simulink model "bo1808_foc_svpwm_bo1808"  (R2024b)
settings: Solver=ode23tb  StartTime=0.0  StopTime=t_stop_position_loop  MaxStep=Ts_sim_foc_svpwm  RelTol=1e-3
PostLoadFcn:
  | try, mf=get_param(bdroot,'FileName'); if ~isempty(mf), addpath(fileparts(fileparts(mf))); end, catch, end
InitFcn:
  | try, mf=get_param(bdroot,'FileName'); if ~isempty(mf), addpath(fileparts(fileparts(mf))); end, catch, end
model workspace (MAT data in the model file):
  B = 5.1285732711e-07
  Id_max = 0.6
  Iq_max = 0.25
  J = 1.4e-07
  Ki_id = 13571.6802635
  Ki_iq = 13571.6802635
  Ki_w = 0.279803284771
  Kp_id = 0.697433569097
  Kp_iq = 0.697433569097
  Kp_pos = 37.6991118431
  Kp_w = 0.0043730736291
  Kt_q = 0.0064
  Ld = 0.00037
  Lq = 0.00037
  Rs = 7.2
  TL_amp_sine = 0.0004
  TL_load_mode = 'step'
  TL_mean_sine = 0.0012
  TL_noise_enable = 0
  TL_noise_sample_time = 0.0001
  TL_noise_seed = 1808
  TL_noise_std = 5e-05
  TL_nom = 0.0012
  TL_sine_start = 0.12
  TL_step_time_fig3_9 = 0.12
  Ts_pwm = 2e-05
  Ts_sim_foc_svpwm = 2e-06
  Vdc = 11.4
  Vdq_max = 6.58179306876
  f_load_sine = 50
  foc_control_mode = 'position'
  omega_ref_pos_max = 104.71975512
  pn = 4
  position_ref_step_time = 0.005
  psi_f = 0.00106666666667
  speed_ref_fig3_9_rpm = 1000
  t_stop_foc_svpwm = 0.25
  t_stop_position_loop = 0.4
  theta_e0 = 0
  theta_m0 = 0
  theta_m_ref_step = 0.523598775598
libraries: simulink x1
settings Model: Creator=26683  LastModifiedBy=26683

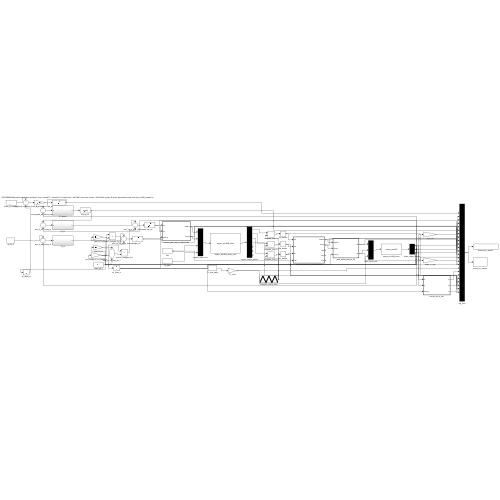
[thumbnail: Simulink's stored preview of the top-level diagram]
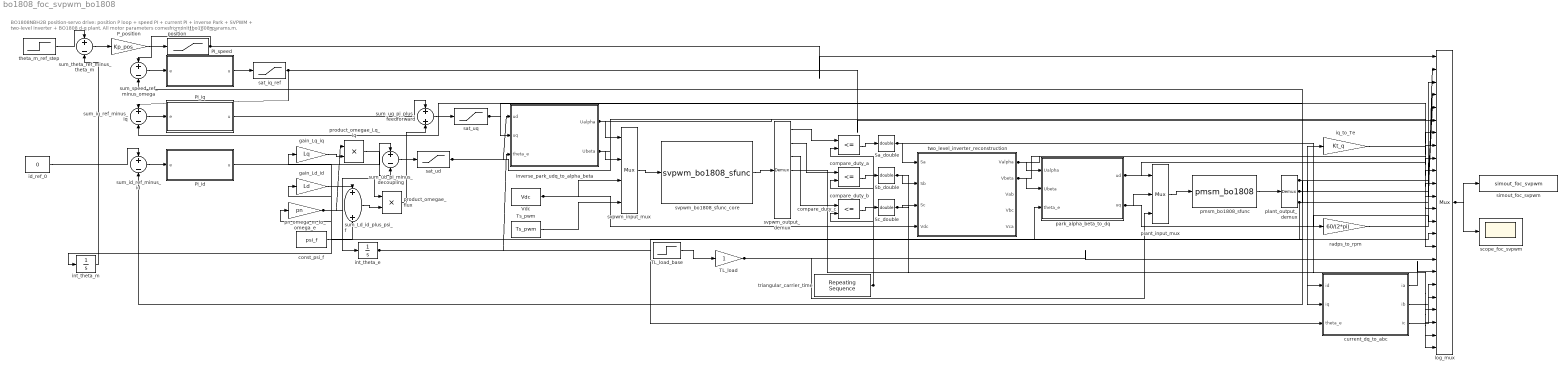
== system bo1808_foc_svpwm_bo1808 ==
  note: BO1808NBH2B position-servo drive: position P loop + speed PI + current PI + inverse Park + SVPWM + two-level inverter + BO1808 d-q plant. All motor parameters come from init_bo1808_params.m.
  PI_id : Subsystem
  PI_iq : Subsystem
  PI_speed : Subsystem
  P_position : Gain  Gain=Kp_pos
  Sa_double : DataTypeConversion  OutDataTypeStr=double  SaturateOnIntegerOverflow=off  RndMeth=Floor
  Sb_double : DataTypeConversion  OutDataTypeStr=double  SaturateOnIntegerOverflow=off  RndMeth=Floor
  Sc_double : DataTypeConversion  OutDataTypeStr=double  SaturateOnIntegerOverflow=off  RndMeth=Floor
  TL_load : Gain
  TL_load_base : Step  Time=TL_step_time_fig3_9  After=TL_nom  SampleTime=0
  Ts_pwm : Constant  Value=Ts_pwm
  Vdc : Constant  Value=Vdc
  compare_duty_a : RelationalOperator  Operator=<=  OutDataTypeStr=boolean  RndMeth=Simplest  InputSameDT=off
  compare_duty_b : RelationalOperator  Operator=<=  OutDataTypeStr=boolean  RndMeth=Simplest  InputSameDT=off
  compare_duty_c : RelationalOperator  Operator=<=  OutDataTypeStr=boolean  RndMeth=Simplest  InputSameDT=off
  const_psi_f : Constant  Value=psi_f
  current_dq_to_abc : MATLAB Function  TreatAsAtomicUnit=on
  gain_Ld_id : Gain  Gain=Ld
  gain_Lq_iq : Gain  Gain=Lq
  id_ref_0 : Constant  Value=0
  int_theta_e : Integrator  InitialCondition=theta_e0
  int_theta_m : Integrator  InitialCondition=theta_m0
  inverse_park_udq_to_alpha_beta : MATLAB Function  TreatAsAtomicUnit=on
  iq_to_Te : Gain  Gain=Kt_q
  log_mux : Mux  Inputs=24
  park_alpha_beta_to_dq : MATLAB Function  TreatAsAtomicUnit=on
  plant_input_mux : Mux  Inputs=3
  plant_output_demux : Demux  Outputs=3
  pmsm_bo1808_sfunc : S-Function  FunctionName=pmsm_bo1808  SFunctionDeploymentMode=off  EnableBusSupport=off
  pn_omega_m_to_omega_e : Gain  Gain=pn
  product_omegae_Lq_iq : Product  Inputs=**
  product_omegae_flux : Product  Inputs=**
  radps_to_rpm : Gain  Gain=60/(2*pi)
  sat_iq_ref : Saturate  UpperLimit=Iq_max  LowerLimit=-Iq_max
  sat_speed_ref_from_position : Saturate  UpperLimit=omega_ref_pos_max  LowerLimit=-omega_ref_pos_max
  sat_ud : Saturate  UpperLimit=Vdq_max  LowerLimit=-Vdq_max
  sat_uq : Saturate  UpperLimit=Vdq_max  LowerLimit=-Vdq_max
  scope_foc_svpwm : Scope
  simout_foc_svpwm : ToWorkspace  VariableName=simout_foc_svpwm  SaveFormat=Structure With Time  SampleTime=-1
  sum_Ld_id_plus_psi_f : Sum
  sum_id_ref_minus_id : Sum  Inputs=+-
  sum_iq_ref_minus_iq : Sum  Inputs=+-
  sum_speed_ref_minus_omega : Sum  Inputs=+-
  sum_theta_ref_minus_theta_m : Sum  Inputs=+-
  sum_ud_pi_minus_decoupling : Sum  Inputs=+-
  sum_uq_pi_plus_feedforward : Sum
  svpwm_bo1808_sfunc_core : S-Function  FunctionName=svpwm_bo1808_sfunc  SFunctionDeploymentMode=off  EnableBusSupport=off
  svpwm_input_mux : Mux
  svpwm_output_demux : Demux  Outputs=7
  theta_m_ref_step : Step  Time=position_ref_step_time  After=theta_m_ref_step  SampleTime=0
  triangular_carrier_time : simulink/Sources/Repeating Sequence  rep_seq_t=[0 Ts_pwm/2 Ts_pwm]  rep_seq_y=[0 Ts_pwm/2 0]
  two_level_inverter_reconstruction : MATLAB Function  TreatAsAtomicUnit=on
  wires:
  TL_load_base/1 -> TL_load/1
  theta_m_ref_step/1 -> sum_theta_ref_minus_theta_m/1
  sum_theta_ref_minus_theta_m/1 -> P_position/1
  P_position/1 -> sat_speed_ref_from_position/1
  sat_speed_ref_from_position/1 -> sum_speed_ref_minus_omega/1, log_mux/1
  sum_speed_ref_minus_omega/1 -> PI_speed/1(e)
  PI_speed/1(u) -> sat_iq_ref/1
  sat_iq_ref/1 -> sum_iq_ref_minus_iq/1, log_mux/6
  id_ref_0/1 -> sum_id_ref_minus_id/1
  sum_iq_ref_minus_iq/1 -> PI_iq/1(e)
  sum_id_ref_minus_id/1 -> PI_id/1(e)
  PI_id/1(u) -> sum_ud_pi_minus_decoupling/1
  product_omegae_Lq_iq/1 -> sum_ud_pi_minus_decoupling/2
  sum_ud_pi_minus_decoupling/1 -> sat_ud/1
  PI_iq/1(u) -> sum_uq_pi_plus_feedforward/1
  product_omegae_flux/1 -> sum_uq_pi_plus_feedforward/2
  sum_uq_pi_plus_feedforward/1 -> sat_uq/1
  sat_ud/1 -> inverse_park_udq_to_alpha_beta/1(ud), log_mux/7
  sat_uq/1 -> inverse_park_udq_to_alpha_beta/2(uq), log_mux/8
  int_theta_e/1 -> inverse_park_udq_to_alpha_beta/3(theta_e), park_alpha_beta_to_dq/3(theta_e), current_dq_to_abc/3(theta_e), log_mux/15
  inverse_park_udq_to_alpha_beta/1(Ualpha) -> svpwm_input_mux/1, log_mux/9
  inverse_park_udq_to_alpha_beta/2(Ubeta) -> svpwm_input_mux/2, log_mux/10
  Vdc/1 -> svpwm_input_mux/3, two_level_inverter_reconstruction/4(Vdc)
  Ts_pwm/1 -> svpwm_input_mux/4
  svpwm_input_mux/1 -> svpwm_bo1808_sfunc_core/1
  svpwm_bo1808_sfunc_core/1 -> svpwm_output_demux/1
  svpwm_output_demux/1 -> compare_duty_a/1
  svpwm_output_demux/2 -> compare_duty_b/1
  svpwm_output_demux/3 -> compare_duty_c/1
  triangular_carrier_time/1 -> compare_duty_a/2, compare_duty_b/2, compare_duty_c/2
  compare_duty_a/1 -> Sa_double/1
  compare_duty_b/1 -> Sb_double/1
  compare_duty_c/1 -> Sc_double/1
  Sa_double/1 -> two_level_inverter_reconstruction/1(Sa), log_mux/22
  Sb_double/1 -> two_level_inverter_reconstruction/2(Sb), log_mux/23
  Sc_double/1 -> two_level_inverter_reconstruction/3(Sc), log_mux/24
  two_level_inverter_reconstruction/1(Valpha) -> park_alpha_beta_to_dq/1(Ualpha), log_mux/11
  two_level_inverter_reconstruction/2(Vbeta) -> park_alpha_beta_to_dq/2(Ubeta), log_mux/12
  park_alpha_beta_to_dq/1(ud) -> plant_input_mux/1, log_mux/13
  park_alpha_beta_to_dq/2(uq) -> plant_input_mux/2, log_mux/14
  TL_load/1 -> plant_input_mux/3, log_mux/17
  plant_input_mux/1 -> pmsm_bo1808_sfunc/1
  pmsm_bo1808_sfunc/1 -> plant_output_demux/1
  plant_output_demux/1 -> sum_id_ref_minus_id/2, gain_Ld_id/1, current_dq_to_abc/1(id), log_mux/4
  plant_output_demux/2 -> sum_iq_ref_minus_iq/2, iq_to_Te/1, gain_Lq_iq/1, current_dq_to_abc/2(iq), log_mux/5
  plant_output_demux/3 -> sum_speed_ref_minus_omega/2, int_theta_m/1, pn_omega_m_to_omega_e/1, radps_to_rpm/1, log_mux/2
  int_theta_m/1 -> sum_theta_ref_minus_theta_m/2
  pn_omega_m_to_omega_e/1 -> int_theta_e/1, product_omegae_Lq_iq/1, product_omegae_flux/1
  gain_Lq_iq/1 -> product_omegae_Lq_iq/2
  gain_Ld_id/1 -> sum_Ld_id_plus_psi_f/1
  const_psi_f/1 -> sum_Ld_id_plus_psi_f/2
  sum_Ld_id_plus_psi_f/1 -> product_omegae_flux/2
  radps_to_rpm/1 -> log_mux/3
  iq_to_Te/1 -> log_mux/16
  current_dq_to_abc/1(ia) -> log_mux/18
  current_dq_to_abc/2(ib) -> log_mux/19
  current_dq_to_abc/3(ic) -> log_mux/20
  svpwm_output_demux/4 -> log_mux/21
  log_mux/1 -> simout_foc_svpwm/1, scope_foc_svpwm/1

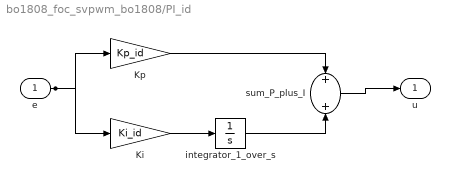
== system bo1808_foc_svpwm_bo1808/PI_id ==
  e : Inport
  Ki : Gain  Gain=Ki_id
  Kp : Gain  Gain=Kp_id
  integrator_1_over_s : Integrator
  sum_P_plus_I : Sum
  u : Outport
  wires:
  e/1 -> Kp/1, Ki/1
  Kp/1 -> sum_P_plus_I/1
  Ki/1 -> integrator_1_over_s/1
  integrator_1_over_s/1 -> sum_P_plus_I/2
  sum_P_plus_I/1 -> u/1

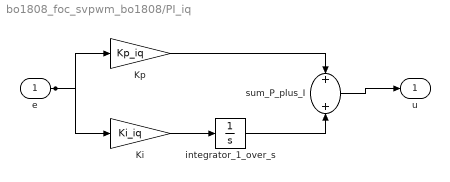
== system bo1808_foc_svpwm_bo1808/PI_iq ==
  e : Inport
  Ki : Gain  Gain=Ki_iq
  Kp : Gain  Gain=Kp_iq
  integrator_1_over_s : Integrator
  sum_P_plus_I : Sum
  u : Outport
  wires:
  e/1 -> Kp/1, Ki/1
  Kp/1 -> sum_P_plus_I/1
  Ki/1 -> integrator_1_over_s/1
  integrator_1_over_s/1 -> sum_P_plus_I/2
  sum_P_plus_I/1 -> u/1

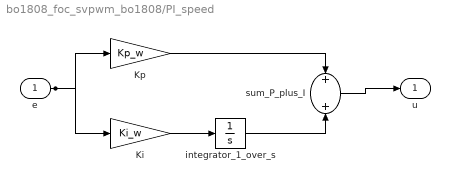
== system bo1808_foc_svpwm_bo1808/PI_speed ==
  e : Inport
  Ki : Gain  Gain=Ki_w
  Kp : Gain  Gain=Kp_w
  integrator_1_over_s : Integrator
  sum_P_plus_I : Sum
  u : Outport
  wires:
  e/1 -> Kp/1, Ki/1
  Kp/1 -> sum_P_plus_I/1
  Ki/1 -> integrator_1_over_s/1
  integrator_1_over_s/1 -> sum_P_plus_I/2
  sum_P_plus_I/1 -> u/1

== matlab function bo1808_foc_svpwm_bo1808/two_level_inverter_reconstruction ==
  data: Sa input; Valpha output; Sb input; Sc input; Vdc input; Vbeta output; Vab output; Vbc output; Vca output
function [Valpha,Vbeta,Vab,Vbc,Vca] = fcn(Sa,Sb,Sc,Vdc)
%#codegen
sa = double(Sa);
sb = double(Sb);
sc = double(Sc);
Va0 = (sa - 0.5)*Vdc;
Vb0 = (sb - 0.5)*Vdc;
Vc0 = (sc - 0.5)*Vdc;
Vab = Va0 - Vb0;
Vbc = Vb0 - Vc0;
Vca = Vc0 - Va0;
Valpha = (2/3)*(Va0 - 0.5*Vb0 - 0.5*Vc0);
Vbeta = (2/3)*(sqrt(3)/2)*(Vb0 - Vc0);
end

== matlab function bo1808_foc_svpwm_bo1808/inverse_park_udq_to_alpha_beta ==
  data: ud input; Ualpha output; uq input; theta_e input; Ubeta output
function [Ualpha,Ubeta] = fcn(ud,uq,theta_e)
%#codegen
c = cos(theta_e);
s = sin(theta_e);
Ualpha = ud*c - uq*s;
Ubeta = ud*s + uq*c;
end

== matlab function bo1808_foc_svpwm_bo1808/park_alpha_beta_to_dq ==
  data: Ualpha input; ud output; Ubeta input; theta_e input; uq output
function [ud,uq] = fcn(Ualpha,Ubeta,theta_e)
%#codegen
c = cos(theta_e);
s = sin(theta_e);
ud = Ualpha*c + Ubeta*s;
uq = -Ualpha*s + Ubeta*c;
end

== matlab function bo1808_foc_svpwm_bo1808/current_dq_to_abc ==
  data: id input; ia output; iq input; theta_e input; ib output; ic output
function [ia,ib,ic] = fcn(id,iq,theta_e)
%#codegen
c = cos(theta_e);
s = sin(theta_e);
ialpha = id*c - iq*s;
ibeta = id*s + iq*c;
ia = ialpha;
ib = -0.5*ialpha + sqrt(3)/2*ibeta;
ic = -0.5*ialpha - sqrt(3)/2*ibeta;
end
